simulink model "W06_S1"  (R2024b)
settings: Solver=ode4  StartTime=0  StopTime=T_final  FixedStep=h  RelTol=1e-3
undefined symbols (not defined in the file or in its folder): beta_c, fit_mode, k_neg, k_pos, mp, N_SEQ, rp, T_max, T_min, T_SW, V_c, x0, X_SEQ, y_pont
settings Model: Creator=admin  LastModifiedBy=admin
settings DataIOCC: ReturnWorkspaceOutputs=off

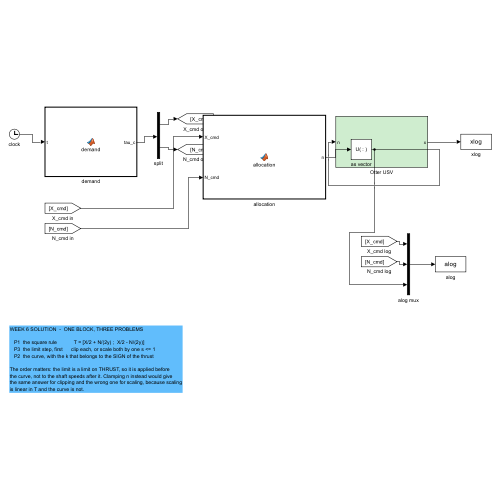
[thumbnail: Simulink's stored preview of the top-level diagram]
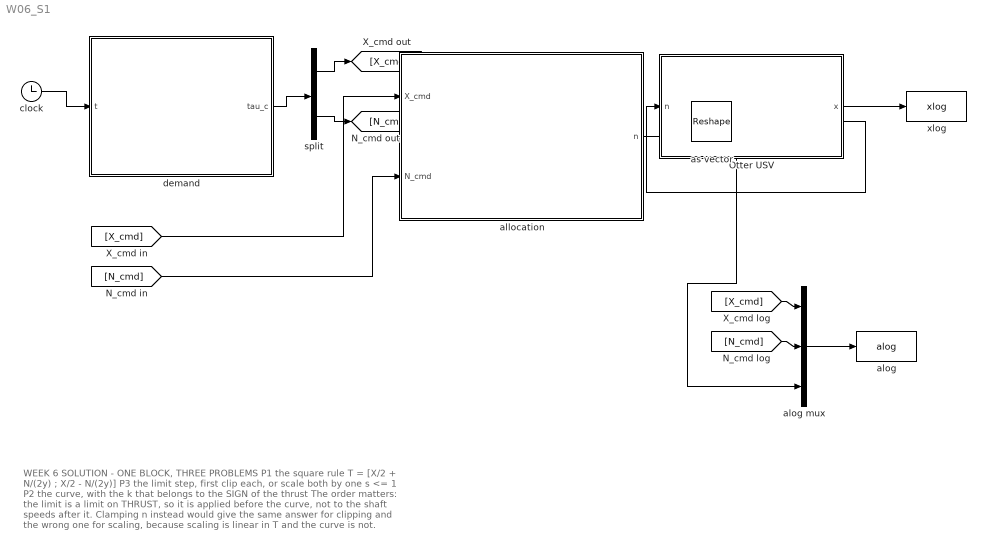
== system W06_S1 ==
  note: WEEK 6 SOLUTION  -  ONE BLOCK, THREE PROBLEMS
      |
      |    P1  the square rule            T = [X/2 + N/(2y) ;  X/2 - N/(2y)]
      |    P3  the limit step, first      clip each, or scale both by one s <= 1
      |    P2  the curve, with the k that belongs to the SIGN of the thrust
      |
      | The order matters: the limit is a limit on THRUST, so it is applied before
      | the curve, not to the shaft speeds after it. Clamping n instead would give
      | the same answer for clipping and the wrong one for scaling, because scaling
      | is linear in T and the curve is not.
  Otter USV : Subsystem
  allocation : MATLAB Function  TreatAsAtomicUnit=on
  alog : ToWorkspace  VariableName=alog  SaveFormat=Structure With Time  SampleTime=-1
  alog mux : Mux  Inputs=3
  as vector : Reshape
  clock : Clock
  demand : MATLAB Function  TreatAsAtomicUnit=on
  split : Demux  Outputs=2
  xlog : ToWorkspace  VariableName=xlog  SaveFormat=Structure With Time  SampleTime=-1
  wires:
  clock/1 -> demand/1(t)
  demand/1(tau_c) -> split/1
  split/1 -> [X_cmd]
  split/2 -> [N_cmd]
  Otter USV/1(x) -> xlog/1
  [X_cmd] -> allocation/1(X_cmd)
  [N_cmd] -> allocation/2(N_cmd)
  allocation/1(n) -> as vector/1
  as vector/1 -> Otter USV/1(n), alog mux/3
  [X_cmd] -> alog mux/1
  [N_cmd] -> alog mux/2
  alog mux/1 -> alog/1

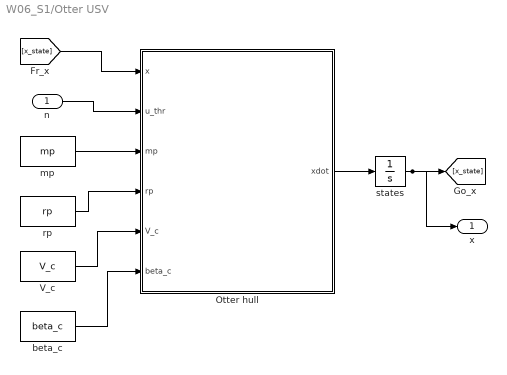
== system W06_S1/Otter USV ==
  n : Inport
  Otter hull : MATLAB Function  TreatAsAtomicUnit=on
  V_c : Constant  Value=V_c
  beta_c : Constant  Value=beta_c
  mp : Constant  Value=mp
  rp : Constant  Value=rp
  states : Integrator  InitialCondition=x0
  x : Outport
  wires:
  mp/1 -> Otter hull/3(mp)
  [x_state] -> Otter hull/1(x)
  n/1 -> Otter hull/2(u_thr)
  rp/1 -> Otter hull/4(rp)
  states/1 -> [x_state], x/1
  V_c/1 -> Otter hull/5(V_c)
  Otter hull/1(xdot) -> states/1
  beta_c/1 -> Otter hull/6(beta_c)

== matlab function W06_S1/Otter USV/Otter hull ==
  data: x input; xdot output double size=[12 1]; u_thr input; mp input; rp input; V_c input; beta_c input
function xdot = otter_hull(x, u_thr, mp, rp, V_c, beta_c)
% Fossen's otter.m, called unchanged from Tools/MSS/VESSELS.
%
%   x       12 states, fed back from the integrator
%   u_thr   propeller shaft speeds [rad/s]
%
% otter.m is not written for code generation, so the call is extrinsic and
% xdot has to be pre-sized for Simulink to know the output width.
coder.extrinsic('otter');

xdot = zeros(12,1);
xdot = otter(x, u_thr, mp, rp, V_c, beta_c);
end

== matlab function W06_S1/demand ==
  data: t input; tau_c output double size=[2 1]; T_SW parameter; X_SEQ parameter; N_SEQ parameter
function tau_c = demand(t, T_SW, X_SEQ, N_SEQ)
%#codegen
%DEMAND  요구 시간표 / the demand timetable.
%
%  T_SW(i) 초부터 (X_SEQ(i), N_SEQ(i)) 를 요구한다. 세 벡터는 워크스페이스에
%  있고, W06_check 가 문제마다 다시 넣는다.
%  From T_SW(i) seconds the demand is (X_SEQ(i), N_SEQ(i)). The three vectors
%  live in the workspace and W06_check sets them for each problem.
k = 1;
for i = 1:numel(T_SW)
    if t >= T_SW(i), k = i; end
end
tau_c = [X_SEQ(k); N_SEQ(k)];

== matlab function W06_S1/allocation ==
  data: X_cmd input; n output double size=[2 1]; N_cmd input; y_pont parameter; k_pos parameter; k_neg parameter; T_max parameter; T_min parameter; fit_mode parameter
function n = allocation(X_cmd, N_cmd, y_pont, k_pos, k_neg, T_max, T_min, fit_mode)
%#codegen
%ALLOCATION  요구한 힘을 두 축의 회전수로 / a demanded force to two shaft speeds.
%
%  세 단계다. 순서가 내용의 일부다.
%  Three steps, and the order is part of the content.
%
%  ── 1) 제곱 규칙 (문제 1, §6-2) ────────────────────────────────────────
%     X = T1 + T2 와 N = y_pont (T1 - T2) 를 T 에 대해 푼 것뿐이다.
%     게인이 없다. 배분은 제어기가 아니라 **역**이고, 역에는 오차가 없다.
%     Nothing but X = T1 + T2 and N = y_pont(T1 - T2), solved for T. There is
%     no gain here: allocation is an inverse, not a controller, and an inverse
%     has no error to act on.
T1 = X_cmd/2 + N_cmd/(2*y_pont);
T2 = X_cmd/2 - N_cmd/(2*y_pont);
%
%  ── 2) 한계 (문제 3, §6-6) ─────────────────────────────────────────────
%     **곡선보다 먼저** 온다. 한계는 추력의 한계이지 회전수의 한계가 아니다.
%     회전수를 자르면 자르기는 같은 답을 주지만 비율 줄이기는 틀린 답을 준다 —
%     비율은 T 에 대해 선형이고 곡선은 아니기 때문이다.
%     This comes BEFORE the curve. The limit is a limit on thrust. Clamping the
%     shaft speed instead gives the same answer for clipping and the wrong one
%     for scaling, because scaling is linear in T and the curve is not.
if fit_mode == 0
    %  자르기: 각각 따로. 쌍이 달라지므로 **방향이 바뀐다**.
    %  Clipping, one thrust at a time: the pair changes, so the direction turns.
    T1 = min(max(T1, T_min), T_max);
    T2 = min(max(T2, T_min), T_max);
else
    %  비율 줄이기: 둘을 **같은 수**로. X 와 N 이 모두 T 에 선형이므로
    %  둘 다 s 배가 되고 비율 X/N 은 그대로 남는다.
    %  Scaling by one factor: X and N are both linear in T, so both are
    %  multiplied by s and the ratio X/N survives exactly.
    s = 1;
    if T1 > T_max, s = min(s, T_max/T1); end
    if T2 > T_max, s = min(s, T_max/T2); end
    if T1 < T_min, s = min(s, T_min/T1); end
    if T2 < T_min, s = min(s, T_min/T2); end
    T1 = s*T1;  T2 = s*T2;
end
%
%  ── 3) 프로펠러 곡선의 역 (문제 2, §6-5) ───────────────────────────────
%     T = k n |n| 의 역은 n = sign(T) sqrt(|T|/k) 인데, **그 k 가 추력의
%     부호에 속한 k 여야 한다.** 앞으로 갈 때는 두 계수가 같은 답을 주므로
%     이 잘못은 시운전에서 살아남는다. 뒤로 갈 때만 드러난다.
%     The inverse needs the k that belongs to the SIGN of the thrust. Ahead,
%     both coefficients agree, which is why this error survives a sea trial:
%     it shows only when something runs astern.
T = [T1; T2];
n = zeros(2,1);
for i = 1:2
    if T(i) >= 0
        n(i) =  sqrt( T(i) / k_pos);
    else
        n(i) = -sqrt(-T(i) / k_neg);
    end
end
